simulink model "Dynamics"  (R2021b)
settings: Solver=FixedStepAuto  StartTime=0.0  StopTime=1000.0  FixedStep=0.1  RelTol=1e-3
values from neighbouring files (symbols this model uses):
  m_noise = [Re;Re;Re;Re;0.0001*Re;0.0001*Re;0.0001*Re]    [main.m]
  p_noise = [Q;Q;Q;Q;Q;Q;Q]    [main.m]
  Ts = 0.1    [main.m]    (also in myStateTransitionFcn.m)
libraries: simulink x3, sharedtransform x3, sharedTrackingLibrary x1
settings Model: Creator=panch  LastModifiedBy=miche

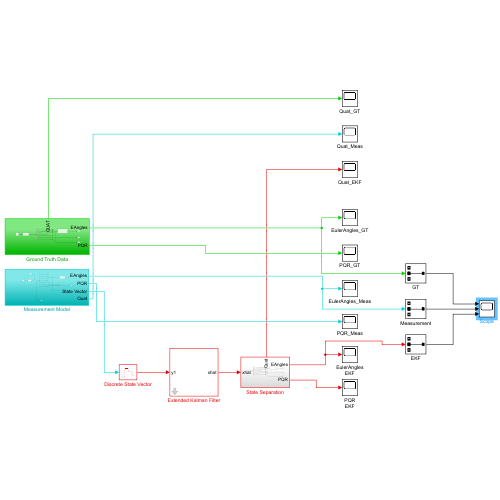
[thumbnail: Simulink's stored preview of the top-level diagram]
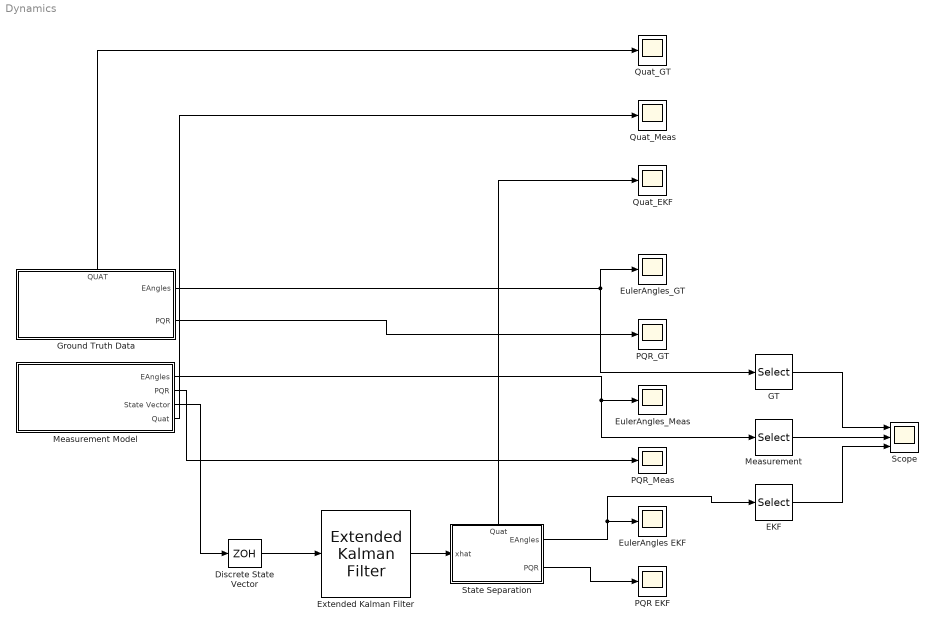
== system Dynamics ==
  Discrete State Vector : ZeroOrderHold  SampleTime=Ts
  EKF : Selector  InputPortWidth=3  IndexOptions=Index vector (dialog)  Indices=2  OutputSizes=1
  EulerAngles EKF : Scope
  EulerAngles_GT : Scope
  EulerAngles_Meas : Scope
  Extended Kalman Filter : sharedTrackingLibrary/Extended Kalman Filter  StateTransitionFcn=myStateTransitionFcn  HasStateTransitionJacobianFcn=off  HasAdditiveProcessNoise=Additive  ProcessNoise=diag(p_noise)  HasTimeVaryingProcessNoise=off  HasStateTransitionFcnExtraArgument=0  InitialState=stateinitial  InitialStateCovariance=1e-16  MeasurementFcn1=myMeasurementFcn  HasMeasurementJacobianFcn1=off  HasMeasurementEnablePort1=off  HasAdditiveMeasurementNoise1=Additive  MeasurementNoise1=diag(m_noise)  HasTimeVaryingMeasurementNoise1=off  HasMeasurementFcnExtraArgument1=0  MeasurementFcn2=myMeasurementFcn  HasMeasurementJacobianFcn2=off  HasMeasurementEnablePort2=off  HasAdditiveMeasurementNoise2=Additive  MeasurementNoise2=1  HasTimeVaryingMeasurementNoise2=off  HasMeasurementFcnExtraArgument2=0  MeasurementFcn3=myMeasurementFcn  HasMeasurementJacobianFcn3=off  HasMeasurementEnablePort3=off  HasAdditiveMeasurementNoise3=Additive  MeasurementNoise3=1  HasTimeVaryingMeasurementNoise3=off  HasMeasurementFcnExtraArgument3=0  MeasurementFcn4=myMeasurementFcn  HasMeasurementJacobianFcn4=off  HasMeasurementEnablePort4=off  HasAdditiveMeasurementNoise4=Additive  MeasurementNoise4=1  HasTimeVaryingMeasurementNoise4=off  HasMeasurementFcnExtraArgument4=0  MeasurementFcn5=myMeasurementFcn  HasMeasurementJacobianFcn5=off  HasMeasurementEnablePort5=off  HasAdditiveMeasurementNoise5=Additive  MeasurementNoise5=1  HasTimeVaryingMeasurementNoise5=off  HasMeasurementFcnExtraArgument5=0  EnableMultirate=off  StateTransitionFcnSampleTime=1  MeasurementFcn1SampleTime=1  MeasurementFcn2SampleTime=1  MeasurementFcn3SampleTime=1  MeasurementFcn4SampleTime=1  MeasurementFcn5SampleTime=1  UseCurrentEstimator=on  OutputStateCovariance=off  DataType=double  SampleTime=Ts  NumberOfMeasurements=1
      settings: SourceProductBaseCode=AE,PW,CT,DR,TF,ID,LP,NV,AR,RO,RR,UV,VE
  GT : Selector  InputPortWidth=3  IndexOptions=Index vector (dialog)  Indices=2  OutputSizes=1
  Ground Truth Data : Subsystem
      settings: PortSchema="{\"entries\":[{\"content\":{\"sides\":[{\"content\":{\"connectorIds\":[]},\"type\":\"ConnectorPlacement.EquallySpacedRectSide\",\"uuid\":\"c56b2d2c-5651-4c6d-ac62-82145f13ec13\"},{\"content\":{\"connectorIds\":[\"Out1\",\"Out2\"],\"side\":\"RIGHT\"},\"type\":\"ConnectorPlacement.EquallySpacedRectSide\",\"uuid\":\"522087ed-b7c5-4ea8-bed0-dd8f980d3eb3\"},{\"content\":{\"connectorIds\":[\"Out3\"],\"side\":\"TOP\"},\"type\":\"ConnectorPlacement.EquallySpacedRectSide\",\"uuid\":\"6b0905f2-79fe-4050-b5fb-9e0d914c666e\"}]},\"type\":\"ConnectorPlacement.EquallySpacedConnector\",\"uuid\":\"925bf434-e85a-4a37-9526-b6377ff21cc2\"}],\"packageUris\":[\"http://schema.mathworks.com/mf0/Connector/R2020b\"],\"version\":\"1.0\"}"
  Measurement : Selector  InputPortWidth=3  IndexOptions=Index vector (dialog)  Indices=2  OutputSizes=1
  Measurement Model : Subsystem
  PQR EKF : Scope
  PQR_GT : Scope
  PQR_Meas : Scope
  Quat_EKF : Scope
  Quat_GT : Scope
  Quat_Meas : Scope
  Scope : Scope  NumInputPorts=3
  State Separation : Subsystem
      settings: PortSchema="{\"entries\":[{\"content\":{\"sides\":[{\"content\":{\"connectorIds\":[\"In1\"]},\"type\":\"ConnectorPlacement.EquallySpacedRectSide\",\"uuid\":\"2e6c3f1f-defd-4c1d-8479-8f40c1cb3474\"},{\"content\":{\"connectorIds\":[\"Out1\",\"Out2\"],\"side\":\"RIGHT\"},\"type\":\"ConnectorPlacement.EquallySpacedRectSide\",\"uuid\":\"64ab90ad-7204-4c28-a9f1-f2fe7aed7ff2\"},{\"content\":{\"connectorIds\":[\"Out3\"],\"side\":\"TOP\"},\"type\":\"ConnectorPlacement.EquallySpacedRectSide\",\"uuid\":\"834626d2-88dc-4687-82b4-c4f469fbfc91\"}]},\"type\":\"ConnectorPlacement.EquallySpacedConnector\",\"uuid\":\"ca35a08a-7abb-4a33-9269-a90c19b82dd3\"}],\"packageUris\":[\"http://schema.mathworks.com/mf0/Connector/R2020b\"],\"version\":\"1.0\"}"
  wires:
  Discrete State Vector/1 -> Extended Kalman Filter/1
  Ground Truth Data/1(EAngles) -> EulerAngles_GT/1, GT/1
  Ground Truth Data/2(PQR) -> PQR_GT/1
  Measurement Model/1(EAngles) -> Measurement/1, EulerAngles_Meas/1
  Measurement Model/2(PQR) -> PQR_Meas/1
  Measurement Model/3(State Vector) -> Discrete State Vector/1
  Extended Kalman Filter/1 -> State Separation/1(xhat)
  State Separation/1(EAngles) -> EKF/1, EulerAngles EKF/1
  State Separation/2(PQR) -> PQR EKF/1
  Measurement/1 -> Scope/2
  GT/1 -> Scope/1
  EKF/1 -> Scope/3
  Ground Truth Data/3(QUAT) -> Quat_GT/1
  Measurement Model/4(Quat) -> Quat_Meas/1
  State Separation/3(Quat) -> Quat_EKF/1

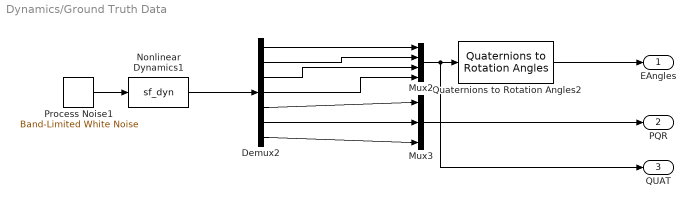
== system Dynamics/Ground Truth Data ==
  Demux2 : Demux  Outputs=7
  Mux2 : Mux
  Mux3 : Mux  Inputs=3
  Nonlinear Dynamics1 : S-Function  FunctionName=sf_dyn  SFunctionDeploymentMode=off  EnableBusSupport=off
  Process Noise1 : simulink/Sources/Band-Limited White Noise  Cov=p_noise*Ts*0  Ts=Ts  seed=[23341]  VectorParams1D=off
  Quaternions to Rotation Angles2 : sharedtransform/Quaternions to Rotation Angles  rotationOrder=ZYX  aMode=aMode
      settings: SourceProductBaseCode=AE,PW,DR,MT,UV,VE
  EAngles : Outport
  PQR : Outport  Port=2
  QUAT : Outport  Port=3
  wires:
  Mux2/1 -> QUAT/1, Quaternions to Rotation Angles2/1
  Process Noise1/1 -> Nonlinear Dynamics1/1
  Nonlinear Dynamics1/1 -> Demux2/1
  Demux2/1 -> Mux2/1
  Demux2/3 -> Mux2/3
  Demux2/2 -> Mux2/2
  Demux2/7 -> Mux3/3
  Demux2/4 -> Mux2/4
  Demux2/6 -> Mux3/2
  Demux2/5 -> Mux3/1
  Quaternions to Rotation Angles2/1 -> EAngles/1
  Mux3/1 -> PQR/1

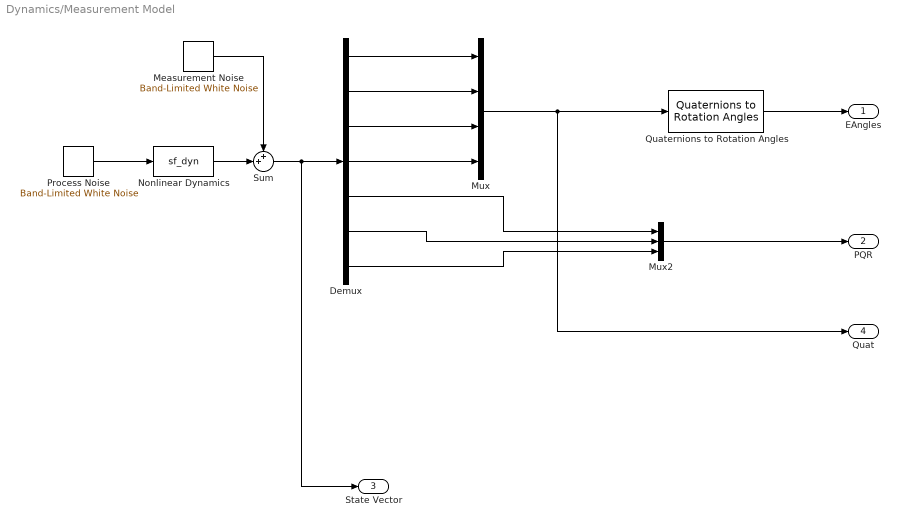
== system Dynamics/Measurement Model ==
  Demux : Demux  Outputs=7
  Measurement Noise : simulink/Sources/Band-Limited White Noise  Cov=500*m_noise*Ts  Ts=Ts  seed=[12347]  VectorParams1D=off
  Mux : Mux
  Mux2 : Mux  Inputs=3
  Nonlinear Dynamics : S-Function  FunctionName=sf_dyn  SFunctionDeploymentMode=off  EnableBusSupport=off
  Process Noise : simulink/Sources/Band-Limited White Noise  Cov=p_noise*Ts  Ts=Ts  seed=[23341]  VectorParams1D=off
  Quaternions to Rotation Angles : sharedtransform/Quaternions to Rotation Angles  rotationOrder=ZYX  aMode=aMode
      settings: SourceProductBaseCode=AE,PW,DR,MT,UV,VE
  Sum : Sum  Inputs=++|
  EAngles : Outport
  PQR : Outport  Port=2
  State Vector : Outport  Port=3
  Quat : Outport  Port=4
  wires:
  Demux/2 -> Mux/2
  Demux/3 -> Mux/3
  Sum/1 -> State Vector/1, Demux/1
  Demux/4 -> Mux/4
  Demux/1 -> Mux/1
  Demux/5 -> Mux2/1
  Demux/7 -> Mux2/3
  Nonlinear Dynamics/1 -> Sum/2
  Mux/1 -> Quat/1, Quaternions to Rotation Angles/1
  Measurement Noise/1 -> Sum/1
  Process Noise/1 -> Nonlinear Dynamics/1
  Demux/6 -> Mux2/2
  Quaternions to Rotation Angles/1 -> EAngles/1
  Mux2/1 -> PQR/1

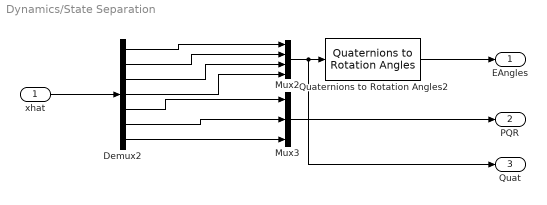
== system Dynamics/State Separation ==
  xhat : Inport
  Demux2 : Demux  Outputs=7
  Mux2 : Mux
  Mux3 : Mux  Inputs=3
  Quaternions to Rotation Angles2 : sharedtransform/Quaternions to Rotation Angles  rotationOrder=ZYX  aMode=aMode
      settings: SourceProductBaseCode=AE,PW,DR,MT,UV,VE
  EAngles : Outport
  PQR : Outport  Port=2
  Quat : Outport  Port=3
  wires:
  Demux2/2 -> Mux2/2
  Demux2/5 -> Mux3/1
  Demux2/6 -> Mux3/2
  Demux2/1 -> Mux2/1
  Demux2/7 -> Mux3/3
  Mux2/1 -> Quat/1, Quaternions to Rotation Angles2/1
  Demux2/3 -> Mux2/3
  Demux2/4 -> Mux2/4
  Mux3/1 -> PQR/1
  xhat/1 -> Demux2/1
  Quaternions to Rotation Angles2/1 -> EAngles/1
